simulink model "Circuit1"  (R2015a)
settings: Solver=ode45  StartTime=0.0  StopTime=10.0  RelTol=1e-3
settings Model: Creator=ROOT  LastModifiedBy=ROOT

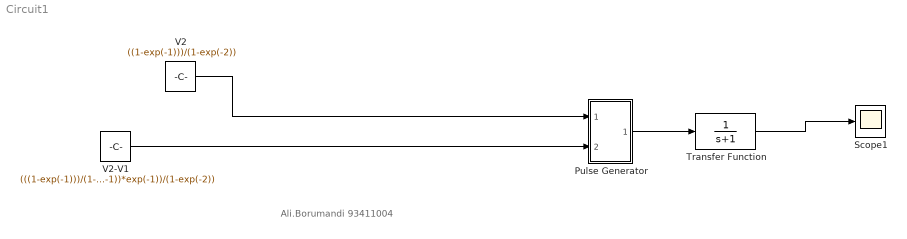
== system Circuit1 ==
  note: Ali.Borumandi 93411004
  Pulse Generator : Subsystem
  Scope1 : Scope
      settings: TickLabels=on  TimeRange=16  YMin=-1  YMax=2
  Transfer Function : TransferFcn  Denominator=[1 1]
  V2 : Constant  Value=((1-exp(-1)))/(1-exp(-2))
  V2-V1 : Constant  Value=(((1-exp(-1)))/(1-exp(-2)))-((1-exp(-1))*exp(-1))/(1-exp(-2))
  wires:
  Transfer Function/1 -> Scope1/1
  V2/1 -> Pulse Generator/1(In1)
  V2-V1/1 -> Pulse Generator/2(In2)
  Pulse Generator/1(Out1) -> Transfer Function/1

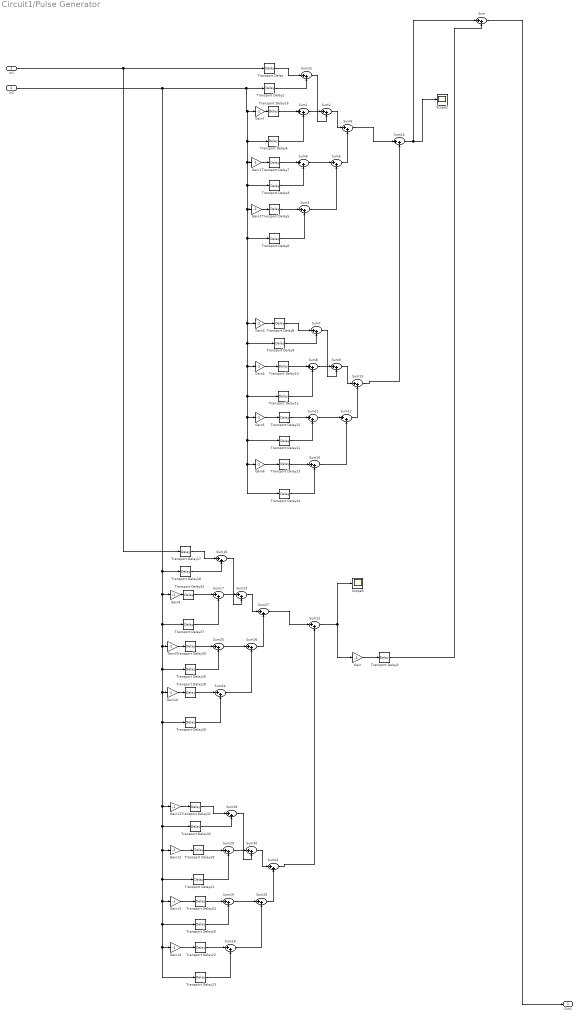
== system Circuit1/Pulse Generator ==
  In1 : Inport
  In2 : Inport  Port=2
  Gain{,1..14} (15 alike) : Gain  Gain=-1
  Scope2 : Scope
      settings: TimeRange=16  YMin=-1  YMax=2
  Scope3 : Scope
      settings: TimeRange=16  YMin=-1  YMax=2
  Sum{,1..30} (31 alike) : Sum  Inputs=|++
  Transport Delay : TransportDelay  DelayTime=0
  Transport Delay1 : TransportDelay
  Transport Delay10 : TransportDelay  DelayTime=10
  Transport Delay11 : TransportDelay  DelayTime=13
  Transport Delay12 : TransportDelay  DelayTime=11
  Transport Delay13 : TransportDelay  DelayTime=14
  Transport Delay14 : TransportDelay  DelayTime=16
  Transport Delay15 : TransportDelay  DelayTime=12
  Transport Delay16 : TransportDelay  DelayTime=2
  Transport Delay17 : TransportDelay  DelayTime=0
  Transport Delay18 : TransportDelay
  Transport Delay19 : TransportDelay  DelayTime=10
  Transport Delay2 : TransportDelay  DelayTime=16
  Transport Delay20 : TransportDelay  DelayTime=13
  Transport Delay21 : TransportDelay  DelayTime=11
  Transport Delay22 : TransportDelay  DelayTime=14
  Transport Delay23 : TransportDelay  DelayTime=16
  Transport Delay24 : TransportDelay  DelayTime=12
  Transport Delay25 : TransportDelay  DelayTime=2
  Transport Delay26 : TransportDelay  DelayTime=5
  Transport Delay27 : TransportDelay  DelayTime=3
  Transport Delay28 : TransportDelay  DelayTime=6
  Transport Delay29 : TransportDelay  DelayTime=7
  Transport Delay3 : TransportDelay  DelayTime=5
  Transport Delay30 : TransportDelay  DelayTime=4
  Transport Delay31 : TransportDelay  DelayTime=8
  Transport Delay32 : TransportDelay  DelayTime=9
  Transport Delay4 : TransportDelay  DelayTime=3
  Transport Delay5 : TransportDelay  DelayTime=6
  Transport Delay6 : TransportDelay  DelayTime=7
  Transport Delay7 : TransportDelay  DelayTime=4
  Transport Delay8 : TransportDelay  DelayTime=8
  Transport Delay9 : TransportDelay  DelayTime=9
  Out1 : Outport
  wires:
  Sum30/1 -> Sum21/1
  Transport Delay20/1 -> Sum19/2
  In1/1 -> Transport Delay17/1, Transport Delay/1
  Transport Delay17/1 -> Sum16/1
  Transport Delay18/1 -> Sum16/2
  Sum16/1 -> Sum23/2
  Gain8/1 -> Transport Delay25/1
  Gain9/1 -> Transport Delay30/1
  Gain10/1 -> Transport Delay28/1
  Gain14/1 -> Transport Delay22/1
  Gain13/1 -> Transport Delay24/1
  Gain12/1 -> Transport Delay19/1
  Gain11/1 -> Transport Delay31/1
  In2/1 -> Transport Delay27/1, Gain11/1, Transport Delay23/1, Gain14/1, Transport Delay20/1, Gain13/1, Transport Delay21/1, Gain12/1, Transport Delay32/1, Transport Delay29/1, Gain10/1, Transport Delay26/1, Gain9/1, Gain8/1, Transport Delay18/1, Transport Delay4/1, Gain3/1, Transport Delay14/1, Gain6/1, Transport Delay11/1, Gain5/1, Transport Delay12/1, Gain4/1, Transport Delay9/1, Transport Delay6/1, Gain2/1, Transport Delay3/1, Gain1/1, Gain7/1, Transport Delay1/1
  Sum22/1 -> Gain/1, Scope3/1
  Transport Delay2/1 -> Sum/2
  Gain/1 -> Transport Delay2/1
  Sum14/1 -> Scope2/1, Sum/1
  Sum/1 -> Out1/1
  Transport Delay16/1 -> Sum1/1
  Sum3/1 -> Sum5/2
  Sum5/1 -> Sum6/2
  Sum2/1 -> Sum6/1
  Gain4/1 -> Transport Delay10/1
  Transport Delay4/1 -> Sum1/2
  Sum4/1 -> Sum5/1
  Transport Delay3/1 -> Sum4/2
  Transport Delay7/1 -> Sum4/1
  Transport Delay5/1 -> Sum3/1
  Sum1/1 -> Sum2/1
  Transport Delay6/1 -> Sum3/2
  Sum23/1 -> Sum27/1
  Transport Delay25/1 -> Sum17/1
  Transport Delay27/1 -> Sum17/2
  Sum26/1 -> Sum27/2
  Sum24/1 -> Sum26/2
  Transport Delay29/1 -> Sum24/2
  Transport Delay26/1 -> Sum25/2
  Transport Delay30/1 -> Sum25/1
  Transport Delay28/1 -> Sum24/1
  Sum25/1 -> Sum26/1
  Sum17/1 -> Sum23/1
  Sum9/1 -> Sum13/1
  Transport Delay11/1 -> Sum11/2
  Gain3/1 -> Transport Delay8/1
  Transport Delay/1 -> Sum15/1
  Transport Delay1/1 -> Sum15/2
  Sum15/1 -> Sum2/2
  Gain2/1 -> Transport Delay5/1
  Gain5/1 -> Transport Delay15/1
  Gain6/1 -> Transport Delay13/1
  Sum18/1 -> Sum20/2
  Sum21/1 -> Sum22/2
  Transport Delay22/1 -> Sum18/1
  Transport Delay32/1 -> Sum28/2
  Transport Delay21/1 -> Sum29/2
  Sum29/1 -> Sum30/1
  Transport Delay23/1 -> Sum18/2
  Sum20/1 -> Sum21/2
  Transport Delay24/1 -> Sum19/1
  Sum27/1 -> Sum22/1
  Transport Delay31/1 -> Sum28/1
  Transport Delay19/1 -> Sum29/1
  Sum19/1 -> Sum20/1
  Sum28/1 -> Sum30/2
  Gain1/1 -> Transport Delay7/1
  Gain7/1 -> Transport Delay16/1
  Sum10/1 -> Sum12/2
  Sum13/1 -> Sum14/2
  Transport Delay13/1 -> Sum10/1
  Transport Delay9/1 -> Sum7/2
  Transport Delay12/1 -> Sum8/2
  Sum8/1 -> Sum9/1
  Transport Delay14/1 -> Sum10/2
  Sum12/1 -> Sum13/2
  Transport Delay15/1 -> Sum11/1
  Sum6/1 -> Sum14/1
  Transport Delay8/1 -> Sum7/1
  Transport Delay10/1 -> Sum8/1
  Sum11/1 -> Sum12/1
  Sum7/1 -> Sum9/2
